simulink model "dam"  (R2023a)
settings: Solver=VariableStepAuto  StartTime=0.0  StopTime=0.5  RelTol=1e-3
libraries: dspfdesign x1
settings Model: Creator=tanov  LastModifiedBy=tanov

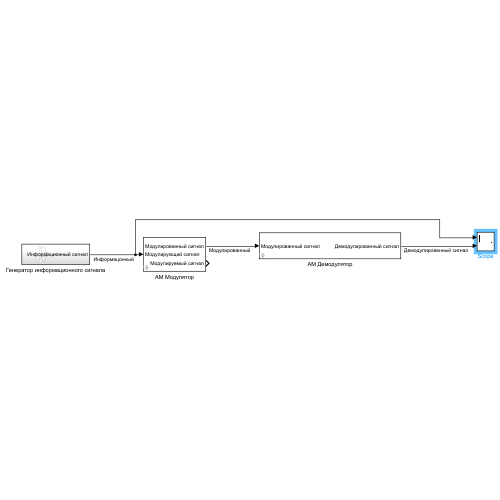
[thumbnail: Simulink's stored preview of the top-level diagram]
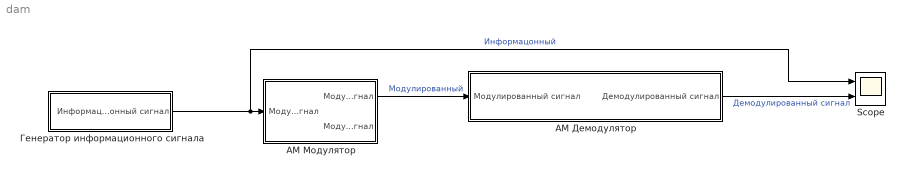
== system dam ==
  AM Демодулятор : Subsystem  mask{f_c=300, m=0.5}
      mask prompts: f_c "Частота несущей"; m "Порядок модуляции"
  AM Модулятор : Subsystem  mask{f_c=300, m=0.5}
      mask prompts: f_c "Частота несущей"; m "Порядок модуляции"
  Scope : Scope  NumInputPorts=2
  Генератор информационного сигнала : Subsystem
  wires:
  Генератор информационного сигнала/1(Информационный сигнал) -> Scope/1, AM Модулятор/1(Модулирующий сигнал)  "Информацонный"
  AM Модулятор/1(Модулированный сигнал) -> AM Демодулятор/1(Модулированный сигнал)  "Модулированный"
  AM Демодулятор/1(Демодулированный сигнал) -> Scope/2  "Демодулированный сигнал"

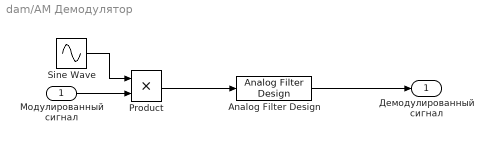
== system dam/AM Демодулятор ==
  Модулированный сигнал : Inport
  Analog Filter Design : dspfdesign/Analog Filter Design  method=Butterworth  filttype=Lowpass  N=16  Wlo=2*pi*f_c  Whi=80  Rp=2  Rs=40
  Product : Product
  Sine Wave : Sin  Frequency=2*pi*f_c  Phase=pi/2  SampleTime=0
  Демодулированный сигнал : Outport
  wires:
  Модулированный сигнал/1 -> Product/2
  Sine Wave/1 -> Product/1
  Product/1 -> Analog Filter Design/1
  Analog Filter Design/1 -> Демодулированный сигнал/1

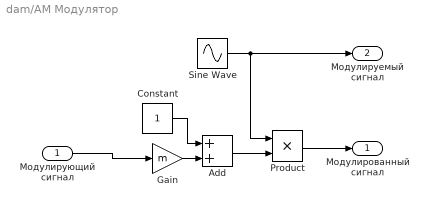
== system dam/AM Модулятор ==
  Модулирующий сигнал : Inport
  Add : Sum
  Constant : Constant
  Gain : Gain  Gain=m
  Product : Product
  Sine Wave : Sin  Frequency=2*pi*f_c  Phase=pi/2  SampleTime=0
  Модулированный сигнал : Outport
  Модулируемый сигнал : Outport  Port=2
  wires:
  Sine Wave/1 -> Product/1, Модулируемый сигнал/1
  Модулирующий сигнал/1 -> Gain/1
  Gain/1 -> Add/2
  Constant/1 -> Add/1
  Add/1 -> Product/2
  Product/1 -> Модулированный сигнал/1

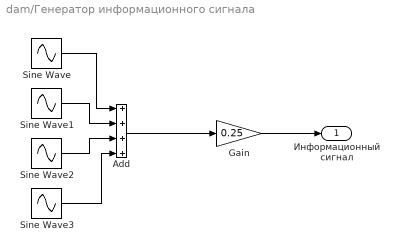
== system dam/Генератор информационного сигнала ==
  Add : Sum  Inputs=++++
  Gain : Gain  Gain=0.25
  Sine Wave : Sin  Frequency=2*pi*40  SampleTime=0
  Sine Wave1 : Sin  Frequency=2*pi*60  SampleTime=0
  Sine Wave2 : Sin  Frequency=2*pi*80  SampleTime=0
  Sine Wave3 : Sin  Frequency=2*pi*100  SampleTime=0
  Информационный сигнал : Outport
  wires:
  Sine Wave/1 -> Add/1
  Sine Wave3/1 -> Add/4
  Sine Wave1/1 -> Add/2
  Sine Wave2/1 -> Add/3
  Add/1 -> Gain/1
  Gain/1 -> Информационный сигнал/1
